simulink model "SPGF_FSK_0000_R2019b"  (R2019b)
settings: Solver=ode3  SolverName=ode4  StartTime=0.0  StopTime=1.4  FixedStep=50e-6/50  RelTol=1e-3  EnableMultiTasking=on
undefined symbols (not defined in the file): D11, Delta
libraries: powerlib x2544, powerlib_meascontrol x204, simulink x24
(part 3 of 33)

== system SPGF_FSK_0000_R2019b/TP21 ==
  Load : powerlib/Elements/Three-Phase Parallel RLC Load  Commented=on  LConnTagsString=A|B|C  Configuration=Y (grounded)  NominalVoltage=380  Vabc=[1e3 1e3 1e3]  Vabcp=[1e3 1e3 1e3]  NominalFrequency=50  UnbalancedPower=off  ActivePower=352800  InductivePower=158760  CapacitivePower=0  Pabc=[10e3 9e3 11e3]  QLabc=[100 90 110]  QCabc=[100 90 110]  Pabcp=[10e3 9e3 11e3]  QLabcp=[100 90 110]  QCabcp=[100 90 110]  Measurements=None  LoadType=constant PQ
  Nonlinear Load : Subsystem  Commented=on
  Nonlinear Load 3ph : Subsystem
  Q : Subsystem
  T : powerlib/Elements/Three-Phase Transformer (Two Windings)  Winding1Connection=Delta (D11)  Winding2Connection=Yg  CoreType=Three single-phase transformers  SetSaturation=on  Hysteresis=off  DataFile='hysteresis'  SetInitialFlux=off  Measurements=None  UNITS=pu  NominalPower=[630000, 50]  Winding1=[10250, 0.00603175, 0.02750000]  Winding2=[400.00, 0.00603175, 0.02750000]  Rm=504  Lm=58.8235  L0=2  Saturation=[0 0;0.01774 0.324129;0.0487637 0.61284;0.0980856 0.825118;0.2 1;0.309543 1.08024;0.652348 1.17344;2.0357 1.26115;6.0215 1.36094;12.4388 1.49469]  InitialFluxes=[-1.05034903009959 0.547738747303872 0.502610282795804]  BreakLoop=on  DiscreteSolver=Trapezoidal iterative  DataType=off  TransfoNumber=1
  Three-Phase Series RLC Load : powerlib/Elements/Three-Phase Series RLC Load  Commented=on  LConnTagsString=A|B|C  Configuration=Y (grounded)  NominalVoltage=380  Vabc=[1e3 1e3 1e3]  Vabcp=[1e3 1e3 1e3]  NominalFrequency=50  UnbalancedPower=off  ActivePower=352800  InductivePower=158760  CapacitivePower=0  Pabc=[10e3 9e3 11e3]  QLabc=[100 90 110]  QCabc=[100 90 110]  Pabcp=[10e3 9e3 11e3]  QLabcp=[100 90 110]  QCabcp=[100 90 110]  Measurements=None  LoadType=constant Z
  Three-Phase Series RLC Load1 : powerlib/Elements/Three-Phase Series RLC Load  LConnTagsString=A|B|C  Configuration=Y (grounded)  NominalVoltage=380  Vabc=[1e3 1e3 1e3]  Vabcp=[1e3 1e3 1e3]  NominalFrequency=50  UnbalancedPower=off  ActivePower=0.1*352800  InductivePower=0  CapacitivePower=0  Pabc=[10e3 9e3 11e3]  QLabc=[100 90 110]  QCabc=[100 90 110]  Pabcp=[10e3 9e3 11e3]  QLabcp=[100 90 110]  QCabcp=[100 90 110]  Measurements=None  LoadType=constant Z
  Three-Phase Series RLC Load2 : powerlib/Elements/Three-Phase Series RLC Load  LConnTagsString=A|B|C  Configuration=Y (grounded)  NominalVoltage=380  Vabc=[1e3 1e3 1e3]  Vabcp=[1e3 1e3 1e3]  NominalFrequency=50  UnbalancedPower=off  ActivePower=0.9*352800  InductivePower=158760  CapacitivePower=0  Pabc=[10e3 9e3 11e3]  QLabc=[100 90 110]  QCabc=[100 90 110]  Pabcp=[10e3 9e3 11e3]  QLabcp=[100 90 110]  QCabcp=[100 90 110]  Measurements=None  LoadType=constant Z
  A : PMIOPort  Side=Right
  B : PMIOPort  Port=2  Side=Right
  C : PMIOPort  Port=3  Side=Right
  connections:
  Three-Phase Series RLC Load/LConn1 -- Nonlinear Load/LConn1 -- Nonlinear Load 3ph/LConn1 -- T/RConn1 -- Load/LConn1 -- Three-Phase Series RLC Load2/LConn1 -- Three-Phase Series RLC Load1/LConn1
  Three-Phase Series RLC Load1/LConn2 -- Three-Phase Series RLC Load2/LConn2 -- Nonlinear Load/LConn2 -- Nonlinear Load 3ph/LConn2 -- Load/LConn2 -- T/RConn2 -- Three-Phase Series RLC Load/LConn2
  Three-Phase Series RLC Load1/LConn3 -- Three-Phase Series RLC Load2/LConn3 -- Nonlinear Load/LConn3 -- Nonlinear Load 3ph/LConn3 -- Load/LConn3 -- T/RConn3 -- Three-Phase Series RLC Load/LConn3
  Q/RConn3 -- C/RConn1
  Q/LConn2 -- T/LConn2
  Q/RConn1 -- A/RConn1
  Q/RConn2 -- B/RConn1
  Q/LConn1 -- T/LConn1
  Q/LConn3 -- T/LConn3

== system SPGF_FSK_0000_R2019b/TP22 ==
  Load : powerlib/Elements/Three-Phase Parallel RLC Load  Commented=on  LConnTagsString=A|B|C  Configuration=Y (grounded)  NominalVoltage=380  Vabc=[1e3 1e3 1e3]  Vabcp=[1e3 1e3 1e3]  NominalFrequency=50  UnbalancedPower=off  ActivePower=352800  InductivePower=158760  CapacitivePower=0  Pabc=[10e3 9e3 11e3]  QLabc=[100 90 110]  QCabc=[100 90 110]  Pabcp=[10e3 9e3 11e3]  QLabcp=[100 90 110]  QCabcp=[100 90 110]  Measurements=None  LoadType=constant PQ
  Nonlinear Load : Subsystem  Commented=on
  Nonlinear Load 3ph : Subsystem
  Q : Subsystem
  T : powerlib/Elements/Three-Phase Transformer (Two Windings)  Winding1Connection=Delta (D11)  Winding2Connection=Yg  CoreType=Three single-phase transformers  SetSaturation=on  Hysteresis=off  DataFile='hysteresis'  SetInitialFlux=off  Measurements=None  UNITS=pu  NominalPower=[630000, 50]  Winding1=[10250, 0.00603175, 0.02750000]  Winding2=[400.00, 0.00603175, 0.02750000]  Rm=504  Lm=58.8235  L0=2  Saturation=[0 0;0.01774 0.324129;0.0487637 0.61284;0.0980856 0.825118;0.2 1;0.309543 1.08024;0.652348 1.17344;2.0357 1.26115;6.0215 1.36094;12.4388 1.49469]  InitialFluxes=[-1.04995444167594 0.547468251609687 0.502486190066125]  BreakLoop=on  DiscreteSolver=Trapezoidal iterative  DataType=off  TransfoNumber=1
  Three-Phase Series RLC Load : powerlib/Elements/Three-Phase Series RLC Load  Commented=on  LConnTagsString=A|B|C  Configuration=Y (grounded)  NominalVoltage=380  Vabc=[1e3 1e3 1e3]  Vabcp=[1e3 1e3 1e3]  NominalFrequency=50  UnbalancedPower=off  ActivePower=352800  InductivePower=158760  CapacitivePower=0  Pabc=[10e3 9e3 11e3]  QLabc=[100 90 110]  QCabc=[100 90 110]  Pabcp=[10e3 9e3 11e3]  QLabcp=[100 90 110]  QCabcp=[100 90 110]  Measurements=None  LoadType=constant Z
  Three-Phase Series RLC Load1 : powerlib/Elements/Three-Phase Series RLC Load  LConnTagsString=A|B|C  Configuration=Y (grounded)  NominalVoltage=380  Vabc=[1e3 1e3 1e3]  Vabcp=[1e3 1e3 1e3]  NominalFrequency=50  UnbalancedPower=off  ActivePower=0.1*352800  InductivePower=0  CapacitivePower=0  Pabc=[10e3 9e3 11e3]  QLabc=[100 90 110]  QCabc=[100 90 110]  Pabcp=[10e3 9e3 11e3]  QLabcp=[100 90 110]  QCabcp=[100 90 110]  Measurements=None  LoadType=constant Z
  Three-Phase Series RLC Load2 : powerlib/Elements/Three-Phase Series RLC Load  LConnTagsString=A|B|C  Configuration=Y (grounded)  NominalVoltage=380  Vabc=[1e3 1e3 1e3]  Vabcp=[1e3 1e3 1e3]  NominalFrequency=50  UnbalancedPower=off  ActivePower=0.9*352800  InductivePower=158760  CapacitivePower=0  Pabc=[10e3 9e3 11e3]  QLabc=[100 90 110]  QCabc=[100 90 110]  Pabcp=[10e3 9e3 11e3]  QLabcp=[100 90 110]  QCabcp=[100 90 110]  Measurements=None  LoadType=constant Z
  A : PMIOPort  Side=Right
  B : PMIOPort  Port=2  Side=Right
  C : PMIOPort  Port=3  Side=Right
  connections:
  Q/LConn3 -- T/LConn3
  Q/LConn1 -- T/LConn1
  Q/RConn2 -- B/RConn1
  Q/RConn1 -- A/RConn1
  Q/LConn2 -- T/LConn2
  Q/RConn3 -- C/RConn1
  Three-Phase Series RLC Load1/LConn3 -- Three-Phase Series RLC Load2/LConn3 -- Nonlinear Load/LConn3 -- Nonlinear Load 3ph/LConn3 -- T/RConn3 -- Load/LConn3 -- Three-Phase Series RLC Load/LConn3
  Three-Phase Series RLC Load1/LConn2 -- Three-Phase Series RLC Load2/LConn2 -- Nonlinear Load/LConn2 -- Nonlinear Load 3ph/LConn2 -- Load/LConn2 -- T/RConn2 -- Three-Phase Series RLC Load/LConn2
  Three-Phase Series RLC Load/LConn1 -- Nonlinear Load/LConn1 -- Nonlinear Load 3ph/LConn1 -- Load/LConn1 -- T/RConn1 -- Three-Phase Series RLC Load2/LConn1 -- Three-Phase Series RLC Load1/LConn1

== system SPGF_FSK_0000_R2019b/TP31 ==
  Load : powerlib/Elements/Three-Phase Parallel RLC Load  Commented=on  LConnTagsString=A|B|C  Configuration=Y (grounded)  NominalVoltage=380  Vabc=[1e3 1e3 1e3]  Vabcp=[1e3 1e3 1e3]  NominalFrequency=50  UnbalancedPower=off  ActivePower=560000  InductivePower=252000  CapacitivePower=0  Pabc=[10e3 9e3 11e3]  QLabc=[100 90 110]  QCabc=[100 90 110]  Pabcp=[10e3 9e3 11e3]  QLabcp=[100 90 110]  QCabcp=[100 90 110]  Measurements=None  LoadType=constant PQ
  Nonlinear Load : Subsystem  Commented=on
  Nonlinear Load 3ph : Subsystem
  Q : Subsystem
  T : powerlib/Elements/Three-Phase Transformer (Two Windings)  Winding1Connection=Y  Winding2Connection=Yg  CoreType=Three single-phase transformers  SetSaturation=on  Hysteresis=off  DataFile='hysteresis'  SetInitialFlux=off  Measurements=None  UNITS=pu  NominalPower=[1000000, 50]  Winding1=[10250, 0.00610000, 0.02750000]  Winding2=[400.00, 0.00610000, 0.02750000]  Rm=526.316  Lm=58.8235  L0=2  Saturation=[0 0;0.01774 0.324129;0.0487637 0.61284;0.0980856 0.825118;0.2 1;0.309543 1.08024;0.652348 1.17344;2.0357 1.26115;6.0215 1.36094;12.4388 1.49469]  InitialFluxes=[-0.919016130821894 0.0257026532083102 0.893313477613749]  BreakLoop=on  DiscreteSolver=Trapezoidal iterative  DataType=off  TransfoNumber=1
  Three-Phase Series RLC Load : powerlib/Elements/Three-Phase Series RLC Load  Commented=on  LConnTagsString=A|B|C  Configuration=Y (grounded)  NominalVoltage=380  Vabc=[1e3 1e3 1e3]  Vabcp=[1e3 1e3 1e3]  NominalFrequency=50  UnbalancedPower=off  ActivePower=560000  InductivePower=252000  CapacitivePower=0  Pabc=[10e3 9e3 11e3]  QLabc=[100 90 110]  QCabc=[100 90 110]  Pabcp=[10e3 9e3 11e3]  QLabcp=[100 90 110]  QCabcp=[100 90 110]  Measurements=None  LoadType=constant Z
  Three-Phase Series RLC Load1 : powerlib/Elements/Three-Phase Series RLC Load  LConnTagsString=A|B|C  Configuration=Y (grounded)  NominalVoltage=380  Vabc=[1e3 1e3 1e3]  Vabcp=[1e3 1e3 1e3]  NominalFrequency=50  UnbalancedPower=off  ActivePower=0.1*560000  InductivePower=0  CapacitivePower=0  Pabc=[10e3 9e3 11e3]  QLabc=[100 90 110]  QCabc=[100 90 110]  Pabcp=[10e3 9e3 11e3]  QLabcp=[100 90 110]  QCabcp=[100 90 110]  Measurements=None  LoadType=constant Z
  Three-Phase Series RLC Load2 : powerlib/Elements/Three-Phase Series RLC Load  LConnTagsString=A|B|C  Configuration=Y (grounded)  NominalVoltage=380  Vabc=[1e3 1e3 1e3]  Vabcp=[1e3 1e3 1e3]  NominalFrequency=50  UnbalancedPower=off  ActivePower=0.9*560000  InductivePower=252000  CapacitivePower=0  Pabc=[10e3 9e3 11e3]  QLabc=[100 90 110]  QCabc=[100 90 110]  Pabcp=[10e3 9e3 11e3]  QLabcp=[100 90 110]  QCabcp=[100 90 110]  Measurements=None  LoadType=constant Z
  A : PMIOPort  Side=Right
  B : PMIOPort  Port=2  Side=Right
  C : PMIOPort  Port=3  Side=Right
  connections:
  Three-Phase Series RLC Load/LConn1 -- Nonlinear Load/LConn1 -- Nonlinear Load 3ph/LConn1 -- T/RConn1 -- Load/LConn1 -- Three-Phase Series RLC Load2/LConn1 -- Three-Phase Series RLC Load1/LConn1
  Three-Phase Series RLC Load1/LConn2 -- Three-Phase Series RLC Load2/LConn2 -- Nonlinear Load/LConn2 -- Nonlinear Load 3ph/LConn2 -- T/RConn2 -- Load/LConn2 -- Three-Phase Series RLC Load/LConn2
  Three-Phase Series RLC Load1/LConn3 -- Three-Phase Series RLC Load2/LConn3 -- Nonlinear Load/LConn3 -- Nonlinear Load 3ph/LConn3 -- T/RConn3 -- Load/LConn3 -- Three-Phase Series RLC Load/LConn3
  Q/RConn3 -- C/RConn1
  Q/LConn2 -- T/LConn2
  Q/RConn1 -- A/RConn1
  Q/RConn2 -- B/RConn1
  Q/LConn1 -- T/LConn1
  Q/LConn3 -- T/LConn3

== system SPGF_FSK_0000_R2019b/TP321 ==
  Load : powerlib/Elements/Three-Phase Parallel RLC Load  Commented=on  LConnTagsString=A|B|C  Configuration=Y (grounded)  NominalVoltage=380  Vabc=[1e3 1e3 1e3]  Vabcp=[1e3 1e3 1e3]  NominalFrequency=50  UnbalancedPower=off  ActivePower=352800  InductivePower=158760  CapacitivePower=0  Pabc=[10e3 9e3 11e3]  QLabc=[100 90 110]  QCabc=[100 90 110]  Pabcp=[10e3 9e3 11e3]  QLabcp=[100 90 110]  QCabcp=[100 90 110]  Measurements=None  LoadType=constant PQ
  Nonlinear Load : Subsystem  Commented=on
  Nonlinear Load 3ph : Subsystem
  Q : Subsystem
  T : powerlib/Elements/Three-Phase Transformer (Two Windings)  Winding1Connection=Delta (D11)  Winding2Connection=Yg  CoreType=Three single-phase transformers  SetSaturation=on  Hysteresis=off  DataFile='hysteresis'  SetInitialFlux=off  Measurements=None  UNITS=pu  NominalPower=[630000, 50]  Winding1=[10250, 0.00603175, 0.02750000]  Winding2=[400.00, 0.00603175, 0.02750000]  Rm=504  Lm=58.8235  L0=2  Saturation=[0 0;0.01774 0.324129;0.0487637 0.61284;0.0980856 0.825118;0.2 1;0.309543 1.08024;0.652348 1.17344;2.0357 1.26115;6.0215 1.36094;12.4388 1.49469]  InitialFluxes=[-1.04481909477767 0.544399254332123 0.500419840445666]  BreakLoop=on  DiscreteSolver=Trapezoidal iterative  DataType=off  TransfoNumber=1
  Three-Phase Series RLC Load : powerlib/Elements/Three-Phase Series RLC Load  Commented=on  LConnTagsString=A|B|C  Configuration=Y (grounded)  NominalVoltage=380  Vabc=[1e3 1e3 1e3]  Vabcp=[1e3 1e3 1e3]  NominalFrequency=50  UnbalancedPower=off  ActivePower=352800  InductivePower=158760  CapacitivePower=0  Pabc=[10e3 9e3 11e3]  QLabc=[100 90 110]  QCabc=[100 90 110]  Pabcp=[10e3 9e3 11e3]  QLabcp=[100 90 110]  QCabcp=[100 90 110]  Measurements=None  LoadType=constant Z
  Three-Phase Series RLC Load1 : powerlib/Elements/Three-Phase Series RLC Load  LConnTagsString=A|B|C  Configuration=Y (grounded)  NominalVoltage=380  Vabc=[1e3 1e3 1e3]  Vabcp=[1e3 1e3 1e3]  NominalFrequency=50  UnbalancedPower=off  ActivePower=0.1*352800  InductivePower=0  CapacitivePower=0  Pabc=[10e3 9e3 11e3]  QLabc=[100 90 110]  QCabc=[100 90 110]  Pabcp=[10e3 9e3 11e3]  QLabcp=[100 90 110]  QCabcp=[100 90 110]  Measurements=None  LoadType=constant Z
  Three-Phase Series RLC Load2 : powerlib/Elements/Three-Phase Series RLC Load  LConnTagsString=A|B|C  Configuration=Y (grounded)  NominalVoltage=380  Vabc=[1e3 1e3 1e3]  Vabcp=[1e3 1e3 1e3]  NominalFrequency=50  UnbalancedPower=off  ActivePower=0.9*352800  InductivePower=158760  CapacitivePower=0  Pabc=[10e3 9e3 11e3]  QLabc=[100 90 110]  QCabc=[100 90 110]  Pabcp=[10e3 9e3 11e3]  QLabcp=[100 90 110]  QCabcp=[100 90 110]  Measurements=None  LoadType=constant Z
  A : PMIOPort  Side=Right
  B : PMIOPort  Port=2  Side=Right
  C : PMIOPort  Port=3  Side=Right
  connections:
  Q/LConn3 -- T/LConn3
  Q/LConn1 -- T/LConn1
  Q/RConn2 -- B/RConn1
  Q/RConn1 -- A/RConn1
  Q/LConn2 -- T/LConn2
  Q/RConn3 -- C/RConn1
  Three-Phase Series RLC Load1/LConn3 -- Three-Phase Series RLC Load2/LConn3 -- Nonlinear Load/LConn3 -- Nonlinear Load 3ph/LConn3 -- T/RConn3 -- Load/LConn3 -- Three-Phase Series RLC Load/LConn3
  Three-Phase Series RLC Load1/LConn2 -- Three-Phase Series RLC Load2/LConn2 -- Nonlinear Load/LConn2 -- Nonlinear Load 3ph/LConn2 -- Load/LConn2 -- T/RConn2 -- Three-Phase Series RLC Load/LConn2
  Three-Phase Series RLC Load/LConn1 -- Nonlinear Load/LConn1 -- Nonlinear Load 3ph/LConn1 -- Load/LConn1 -- T/RConn1 -- Three-Phase Series RLC Load2/LConn1 -- Three-Phase Series RLC Load1/LConn1

== system SPGF_FSK_0000_R2019b/TP322 ==
  Load : powerlib/Elements/Three-Phase Parallel RLC Load  Commented=on  LConnTagsString=A|B|C  Configuration=Y (grounded)  NominalVoltage=380  Vabc=[1e3 1e3 1e3]  Vabcp=[1e3 1e3 1e3]  NominalFrequency=50  UnbalancedPower=off  ActivePower=352800  InductivePower=158760  CapacitivePower=0  Pabc=[10e3 9e3 11e3]  QLabc=[100 90 110]  QCabc=[100 90 110]  Pabcp=[10e3 9e3 11e3]  QLabcp=[100 90 110]  QCabcp=[100 90 110]  Measurements=None  LoadType=constant PQ
  Nonlinear Load : Subsystem  Commented=on
  Nonlinear Load 3ph : Subsystem
  Q : Subsystem
  T : powerlib/Elements/Three-Phase Transformer (Two Windings)  Winding1Connection=Delta (D11)  Winding2Connection=Yg  CoreType=Three single-phase transformers  SetSaturation=on  Hysteresis=off  DataFile='hysteresis'  SetInitialFlux=off  Measurements=None  UNITS=pu  NominalPower=[630000, 50]  Winding1=[10250, 0.00603175, 0.02750000]  Winding2=[400.00, 0.00603175, 0.02750000]  Rm=504  Lm=58.8235  L0=2  Saturation=[0 0;0.01774 0.324129;0.0487637 0.61284;0.0980856 0.825118;0.2 1;0.309543 1.08024;0.652348 1.17344;2.0357 1.26115;6.0215 1.36094;12.4388 1.49469]  InitialFluxes=[-1.0448190947778 0.544399254332092 0.500419840445633]  BreakLoop=on  DiscreteSolver=Trapezoidal iterative  DataType=off  TransfoNumber=1
  Three-Phase Series RLC Load : powerlib/Elements/Three-Phase Series RLC Load  Commented=on  LConnTagsString=A|B|C  Configuration=Y (grounded)  NominalVoltage=380  Vabc=[1e3 1e3 1e3]  Vabcp=[1e3 1e3 1e3]  NominalFrequency=50  UnbalancedPower=off  ActivePower=352800  InductivePower=158760  CapacitivePower=0  Pabc=[10e3 9e3 11e3]  QLabc=[100 90 110]  QCabc=[100 90 110]  Pabcp=[10e3 9e3 11e3]  QLabcp=[100 90 110]  QCabcp=[100 90 110]  Measurements=None  LoadType=constant Z
  Three-Phase Series RLC Load1 : powerlib/Elements/Three-Phase Series RLC Load  LConnTagsString=A|B|C  Configuration=Y (grounded)  NominalVoltage=380  Vabc=[1e3 1e3 1e3]  Vabcp=[1e3 1e3 1e3]  NominalFrequency=50  UnbalancedPower=off  ActivePower=0.1*352800  InductivePower=0  CapacitivePower=0  Pabc=[10e3 9e3 11e3]  QLabc=[100 90 110]  QCabc=[100 90 110]  Pabcp=[10e3 9e3 11e3]  QLabcp=[100 90 110]  QCabcp=[100 90 110]  Measurements=None  LoadType=constant Z
  Three-Phase Series RLC Load2 : powerlib/Elements/Three-Phase Series RLC Load  LConnTagsString=A|B|C  Configuration=Y (grounded)  NominalVoltage=380  Vabc=[1e3 1e3 1e3]  Vabcp=[1e3 1e3 1e3]  NominalFrequency=50  UnbalancedPower=off  ActivePower=0.9*352800  InductivePower=158760  CapacitivePower=0  Pabc=[10e3 9e3 11e3]  QLabc=[100 90 110]  QCabc=[100 90 110]  Pabcp=[10e3 9e3 11e3]  QLabcp=[100 90 110]  QCabcp=[100 90 110]  Measurements=None  LoadType=constant Z
  A : PMIOPort  Side=Right
  B : PMIOPort  Port=2  Side=Right
  C : PMIOPort  Port=3  Side=Right
  connections:
  Three-Phase Series RLC Load/LConn1 -- Nonlinear Load/LConn1 -- Nonlinear Load 3ph/LConn1 -- Load/LConn1 -- T/RConn1 -- Three-Phase Series RLC Load2/LConn1 -- Three-Phase Series RLC Load1/LConn1
  Three-Phase Series RLC Load1/LConn2 -- Three-Phase Series RLC Load2/LConn2 -- Nonlinear Load/LConn2 -- Nonlinear Load 3ph/LConn2 -- T/RConn2 -- Load/LConn2 -- Three-Phase Series RLC Load/LConn2
  Three-Phase Series RLC Load1/LConn3 -- Three-Phase Series RLC Load2/LConn3 -- Nonlinear Load/LConn3 -- Nonlinear Load 3ph/LConn3 -- T/RConn3 -- Load/LConn3 -- Three-Phase Series RLC Load/LConn3
  Q/RConn3 -- C/RConn1
  Q/LConn2 -- T/LConn2
  Q/RConn1 -- A/RConn1
  Q/RConn2 -- B/RConn1
  Q/LConn1 -- T/LConn1
  Q/LConn3 -- T/LConn3

== system SPGF_FSK_0000_R2019b/TP33 ==
  Load : powerlib/Elements/Three-Phase Parallel RLC Load  Commented=on  LConnTagsString=A|B|C  Configuration=Y (grounded)  NominalVoltage=380  Vabc=[1e3 1e3 1e3]  Vabcp=[1e3 1e3 1e3]  NominalFrequency=50  UnbalancedPower=off  ActivePower=560000  InductivePower=252000  CapacitivePower=0  Pabc=[10e3 9e3 11e3]  QLabc=[100 90 110]  QCabc=[100 90 110]  Pabcp=[10e3 9e3 11e3]  QLabcp=[100 90 110]  QCabcp=[100 90 110]  Measurements=None  LoadType=constant PQ
  Nonlinear Load : Subsystem  Commented=on
  Nonlinear Load 3ph : Subsystem
  Q : Subsystem
  T : powerlib/Elements/Three-Phase Transformer (Two Windings)  Winding1Connection=Y  Winding2Connection=Yg  CoreType=Three single-phase transformers  SetSaturation=on  Hysteresis=off  DataFile='hysteresis'  SetInitialFlux=off  Measurements=None  UNITS=pu  NominalPower=[1000000, 50]  Winding1=[10250, 0.00610000, 0.02750000]  Winding2=[400.00, 0.00610000, 0.02750000]  Rm=526.316  Lm=58.8235  L0=2  Saturation=[0 0;0.01774 0.324129;0.0487637 0.61284;0.0980856 0.825118;0.2 1;0.309543 1.08024;0.652348 1.17344;2.0357 1.26115;6.0215 1.36094;12.4388 1.49469]  InitialFluxes=[-0.916567668392243 0.025179277852983 0.891388390539228]  BreakLoop=on  DiscreteSolver=Trapezoidal iterative  DataType=off  TransfoNumber=1
  Three-Phase Series RLC Load : powerlib/Elements/Three-Phase Series RLC Load  Commented=on  LConnTagsString=A|B|C  Configuration=Y (grounded)  NominalVoltage=380  Vabc=[1e3 1e3 1e3]  Vabcp=[1e3 1e3 1e3]  NominalFrequency=50  UnbalancedPower=off  ActivePower=560000  InductivePower=252000  CapacitivePower=0  Pabc=[10e3 9e3 11e3]  QLabc=[100 90 110]  QCabc=[100 90 110]  Pabcp=[10e3 9e3 11e3]  QLabcp=[100 90 110]  QCabcp=[100 90 110]  Measurements=None  LoadType=constant Z
  Three-Phase Series RLC Load1 : powerlib/Elements/Three-Phase Series RLC Load  LConnTagsString=A|B|C  Configuration=Y (grounded)  NominalVoltage=380  Vabc=[1e3 1e3 1e3]  Vabcp=[1e3 1e3 1e3]  NominalFrequency=50  UnbalancedPower=off  ActivePower=0.1*560000  InductivePower=0  CapacitivePower=0  Pabc=[10e3 9e3 11e3]  QLabc=[100 90 110]  QCabc=[100 90 110]  Pabcp=[10e3 9e3 11e3]  QLabcp=[100 90 110]  QCabcp=[100 90 110]  Measurements=None  LoadType=constant Z
  Three-Phase Series RLC Load2 : powerlib/Elements/Three-Phase Series RLC Load  LConnTagsString=A|B|C  Configuration=Y (grounded)  NominalVoltage=380  Vabc=[1e3 1e3 1e3]  Vabcp=[1e3 1e3 1e3]  NominalFrequency=50  UnbalancedPower=off  ActivePower=0.9*560000  InductivePower=252000  CapacitivePower=0  Pabc=[10e3 9e3 11e3]  QLabc=[100 90 110]  QCabc=[100 90 110]  Pabcp=[10e3 9e3 11e3]  QLabcp=[100 90 110]  QCabcp=[100 90 110]  Measurements=None  LoadType=constant Z
  A : PMIOPort  Side=Right
  B : PMIOPort  Port=2  Side=Right
  C : PMIOPort  Port=3  Side=Right
  connections:
  Q/LConn3 -- T/LConn3
  Q/LConn1 -- T/LConn1
  Q/RConn2 -- B/RConn1
  Q/RConn1 -- A/RConn1
  Q/LConn2 -- T/LConn2
  Q/RConn3 -- C/RConn1
  Three-Phase Series RLC Load1/LConn3 -- Three-Phase Series RLC Load2/LConn3 -- Nonlinear Load/LConn3 -- Nonlinear Load 3ph/LConn3 -- T/RConn3 -- Load/LConn3 -- Three-Phase Series RLC Load/LConn3
  Three-Phase Series RLC Load1/LConn2 -- Three-Phase Series RLC Load2/LConn2 -- Nonlinear Load/LConn2 -- Nonlinear Load 3ph/LConn2 -- Load/LConn2 -- T/RConn2 -- Three-Phase Series RLC Load/LConn2
  Three-Phase Series RLC Load/LConn1 -- Nonlinear Load/LConn1 -- Nonlinear Load 3ph/LConn1 -- Load/LConn1 -- T/RConn1 -- Three-Phase Series RLC Load2/LConn1 -- Three-Phase Series RLC Load1/LConn1

== system SPGF_FSK_0000_R2019b/TP34 ==
  Load : powerlib/Elements/Three-Phase Parallel RLC Load  Commented=on  LConnTagsString=A|B|C  Configuration=Y (grounded)  NominalVoltage=380  Vabc=[1e3 1e3 1e3]  Vabcp=[1e3 1e3 1e3]  NominalFrequency=50  UnbalancedPower=off  ActivePower=352800  InductivePower=158760  CapacitivePower=0  Pabc=[10e3 9e3 11e3]  QLabc=[100 90 110]  QCabc=[100 90 110]  Pabcp=[10e3 9e3 11e3]  QLabcp=[100 90 110]  QCabcp=[100 90 110]  Measurements=None  LoadType=constant PQ
  Nonlinear Load : Subsystem  Commented=on
  Nonlinear Load 3ph : Subsystem
  Q : Subsystem
  T : powerlib/Elements/Three-Phase Transformer (Two Windings)  Winding1Connection=Delta (D11)  Winding2Connection=Yg  CoreType=Three single-phase transformers  SetSaturation=on  Hysteresis=off  DataFile='hysteresis'  SetInitialFlux=off  Measurements=None  UNITS=pu  NominalPower=[630000, 50]  Winding1=[10250, 0.00603175, 0.02750000]  Winding2=[400.00, 0.00603175, 0.02750000]  Rm=504  Lm=58.8235  L0=2  Saturation=[0 0;0.01774 0.324129;0.0487637 0.61284;0.0980856 0.825118;0.2 1;0.309543 1.08024;0.652348 1.17344;2.0357 1.26115;6.0215 1.36094;12.4388 1.49469]  InitialFluxes=[-1.04232437769437 0.542559009201154 0.499765368493118]  BreakLoop=on  DiscreteSolver=Trapezoidal iterative  DataType=off  TransfoNumber=1
  Three-Phase Series RLC Load : powerlib/Elements/Three-Phase Series RLC Load  Commented=on  LConnTagsString=A|B|C  Configuration=Y (grounded)  NominalVoltage=380  Vabc=[1e3 1e3 1e3]  Vabcp=[1e3 1e3 1e3]  NominalFrequency=50  UnbalancedPower=off  ActivePower=352800  InductivePower=158760  CapacitivePower=0  Pabc=[10e3 9e3 11e3]  QLabc=[100 90 110]  QCabc=[100 90 110]  Pabcp=[10e3 9e3 11e3]  QLabcp=[100 90 110]  QCabcp=[100 90 110]  Measurements=None  LoadType=constant Z
  Three-Phase Series RLC Load1 : powerlib/Elements/Three-Phase Series RLC Load  LConnTagsString=A|B|C  Configuration=Y (grounded)  NominalVoltage=380  Vabc=[1e3 1e3 1e3]  Vabcp=[1e3 1e3 1e3]  NominalFrequency=50  UnbalancedPower=off  ActivePower=0.1*352800  InductivePower=0  CapacitivePower=0  Pabc=[10e3 9e3 11e3]  QLabc=[100 90 110]  QCabc=[100 90 110]  Pabcp=[10e3 9e3 11e3]  QLabcp=[100 90 110]  QCabcp=[100 90 110]  Measurements=None  LoadType=constant Z
  Three-Phase Series RLC Load2 : powerlib/Elements/Three-Phase Series RLC Load  LConnTagsString=A|B|C  Configuration=Y (grounded)  NominalVoltage=380  Vabc=[1e3 1e3 1e3]  Vabcp=[1e3 1e3 1e3]  NominalFrequency=50  UnbalancedPower=off  ActivePower=0.9*352800  InductivePower=158760  CapacitivePower=0  Pabc=[10e3 9e3 11e3]  QLabc=[100 90 110]  QCabc=[100 90 110]  Pabcp=[10e3 9e3 11e3]  QLabcp=[100 90 110]  QCabcp=[100 90 110]  Measurements=None  LoadType=constant Z
  A : PMIOPort  Side=Right
  B : PMIOPort  Port=2  Side=Right
  C : PMIOPort  Port=3  Side=Right
  connections:
  Three-Phase Series RLC Load2/LConn1 -- Three-Phase Series RLC Load1/LConn1 -- Three-Phase Series RLC Load/LConn1 -- Nonlinear Load/LConn1 -- Nonlinear Load 3ph/LConn1 -- Load/LConn1 -- T/RConn1
  Three-Phase Series RLC Load2/LConn2 -- Three-Phase Series RLC Load1/LConn2 -- Three-Phase Series RLC Load/LConn2 -- Nonlinear Load/LConn2 -- Nonlinear Load 3ph/LConn2 -- Load/LConn2 -- T/RConn2
  Three-Phase Series RLC Load1/LConn3 -- Three-Phase Series RLC Load2/LConn3 -- Three-Phase Series RLC Load/LConn3 -- Load/LConn3 -- T/RConn3 -- Nonlinear Load/LConn3 -- Nonlinear Load 3ph/LConn3
  Q/RConn3 -- C/RConn1
  Q/LConn2 -- T/LConn2
  Q/RConn1 -- A/RConn1
  Q/RConn2 -- B/RConn1
  Q/LConn1 -- T/LConn1
  Q/LConn3 -- T/LConn3

== system SPGF_FSK_0000_R2019b/TP35 ==
  Load : powerlib/Elements/Three-Phase Parallel RLC Load  Commented=on  LConnTagsString=A|B|C  Configuration=Y (grounded)  NominalVoltage=380  Vabc=[1e3 1e3 1e3]  Vabcp=[1e3 1e3 1e3]  NominalFrequency=50  UnbalancedPower=off  ActivePower=224000  InductivePower=100800  CapacitivePower=0  Pabc=[10e3 9e3 11e3]  QLabc=[100 90 110]  QCabc=[100 90 110]  Pabcp=[10e3 9e3 11e3]  QLabcp=[100 90 110]  QCabcp=[100 90 110]  Measurements=None  LoadType=constant PQ
  Nonlinear Load : Subsystem  Commented=on
  Nonlinear Load 3ph : Subsystem
  Q : Subsystem
  T : powerlib/Elements/Three-Phase Transformer (Two Windings)  Winding1Connection=Y  Winding2Connection=Yg  CoreType=Three single-phase transformers  SetSaturation=on  Hysteresis=off  DataFile='hysteresis'  SetInitialFlux=off  Measurements=None  UNITS=pu  NominalPower=[400000, 50]  Winding1=[10250, 0.00687500, 0.02250000]  Winding2=[400.00, 0.00687500, 0.02250000]  Rm=444.444  Lm=55.5556  L0=2  Saturation=[0 0;0.01774 0.324129;0.0487637 0.61284;0.0980856 0.825118;0.2 1;0.309543 1.08024;0.652348 1.17344;2.0357 1.26115;6.0215 1.36094;12.4388 1.49469]  InitialFluxes=[-0.913549221158618 0.0211591996653002 0.892390021493428]  BreakLoop=on  DiscreteSolver=Trapezoidal iterative  DataType=off  TransfoNumber=1
  Three-Phase Series RLC Load : powerlib/Elements/Three-Phase Series RLC Load  Commented=on  LConnTagsString=A|B|C  Configuration=Y (grounded)  NominalVoltage=380  Vabc=[1e3 1e3 1e3]  Vabcp=[1e3 1e3 1e3]  NominalFrequency=50  UnbalancedPower=off  ActivePower=224000  InductivePower=100800  CapacitivePower=0  Pabc=[10e3 9e3 11e3]  QLabc=[100 90 110]  QCabc=[100 90 110]  Pabcp=[10e3 9e3 11e3]  QLabcp=[100 90 110]  QCabcp=[100 90 110]  Measurements=None  LoadType=constant Z
  Three-Phase Series RLC Load1 : powerlib/Elements/Three-Phase Series RLC Load  LConnTagsString=A|B|C  Configuration=Y (grounded)  NominalVoltage=380  Vabc=[1e3 1e3 1e3]  Vabcp=[1e3 1e3 1e3]  NominalFrequency=50  UnbalancedPower=off  ActivePower=0.1*224000  InductivePower=0  CapacitivePower=0  Pabc=[10e3 9e3 11e3]  QLabc=[100 90 110]  QCabc=[100 90 110]  Pabcp=[10e3 9e3 11e3]  QLabcp=[100 90 110]  QCabcp=[100 90 110]  Measurements=None  LoadType=constant Z
  Three-Phase Series RLC Load2 : powerlib/Elements/Three-Phase Series RLC Load  LConnTagsString=A|B|C  Configuration=Y (grounded)  NominalVoltage=380  Vabc=[1e3 1e3 1e3]  Vabcp=[1e3 1e3 1e3]  NominalFrequency=50  UnbalancedPower=off  ActivePower=0.9*224000  InductivePower=100800  CapacitivePower=0  Pabc=[10e3 9e3 11e3]  QLabc=[100 90 110]  QCabc=[100 90 110]  Pabcp=[10e3 9e3 11e3]  QLabcp=[100 90 110]  QCabcp=[100 90 110]  Measurements=None  LoadType=constant Z
  A : PMIOPort  Side=Right
  B : PMIOPort  Port=2  Side=Right
  C : PMIOPort  Port=3  Side=Right
  connections:
  Q/LConn3 -- T/LConn3
  Q/LConn1 -- T/LConn1
  Q/RConn2 -- B/RConn1
  Q/RConn1 -- A/RConn1
  Q/LConn2 -- T/LConn2
  Q/RConn3 -- C/RConn1
  Three-Phase Series RLC Load1/LConn3 -- Three-Phase Series RLC Load2/LConn3 -- Nonlinear Load/LConn3 -- Nonlinear Load 3ph/LConn3 -- T/RConn3 -- Load/LConn3 -- Three-Phase Series RLC Load/LConn3
  Three-Phase Series RLC Load1/LConn2 -- Three-Phase Series RLC Load2/LConn2 -- Nonlinear Load/LConn2 -- Nonlinear Load 3ph/LConn2 -- T/RConn2 -- Load/LConn2 -- Three-Phase Series RLC Load/LConn2
  Three-Phase Series RLC Load/LConn1 -- Nonlinear Load/LConn1 -- Nonlinear Load 3ph/LConn1 -- Load/LConn1 -- T/RConn1 -- Three-Phase Series RLC Load2/LConn1 -- Three-Phase Series RLC Load1/LConn1

== system SPGF_FSK_0000_R2019b/TP41 ==
  Load : powerlib/Elements/Three-Phase Parallel RLC Load  Commented=on  LConnTagsString=A|B|C  Configuration=Y (grounded)  NominalVoltage=380  Vabc=[1e3 1e3 1e3]  Vabcp=[1e3 1e3 1e3]  NominalFrequency=50  UnbalancedPower=off  ActivePower=352800  InductivePower=158760  CapacitivePower=0  Pabc=[10e3 9e3 11e3]  QLabc=[100 90 110]  QCabc=[100 90 110]  Pabcp=[10e3 9e3 11e3]  QLabcp=[100 90 110]  QCabcp=[100 90 110]  Measurements=None  LoadType=constant PQ
  Nonlinear Load : Subsystem  Commented=on
  Nonlinear Load 3ph : Subsystem
  Q : Subsystem
  T : powerlib/Elements/Three-Phase Transformer (Two Windings)  Winding1Connection=Delta (D11)  Winding2Connection=Yg  CoreType=Three single-phase transformers  SetSaturation=on  Hysteresis=off  DataFile='hysteresis'  SetInitialFlux=off  Measurements=None  UNITS=pu  NominalPower=[630000, 50]  Winding1=[10250, 0.00603175, 0.02750000]  Winding2=[400.00, 0.00603175, 0.02750000]  Rm=504  Lm=58.8235  L0=2  Saturation=[0 0;0.01774 0.324129;0.0487637 0.61284;0.0980856 0.825118;0.2 1;0.309543 1.08024;0.652348 1.17344;2.0357 1.26115;6.0215 1.36094;12.4388 1.49469]  InitialFluxes=[-1.0503661048076 0.547751977522492 0.502614127285616]  BreakLoop=on  DiscreteSolver=Trapezoidal iterative  DataType=off  TransfoNumber=1
  Three-Phase Series RLC Load : powerlib/Elements/Three-Phase Series RLC Load  Commented=on  LConnTagsString=A|B|C  Configuration=Y (grounded)  NominalVoltage=380  Vabc=[1e3 1e3 1e3]  Vabcp=[1e3 1e3 1e3]  NominalFrequency=50  UnbalancedPower=off  ActivePower=352800  InductivePower=158760  CapacitivePower=0  Pabc=[10e3 9e3 11e3]  QLabc=[100 90 110]  QCabc=[100 90 110]  Pabcp=[10e3 9e3 11e3]  QLabcp=[100 90 110]  QCabcp=[100 90 110]  Measurements=None  LoadType=constant Z
  Three-Phase Series RLC Load1 : powerlib/Elements/Three-Phase Series RLC Load  LConnTagsString=A|B|C  Configuration=Y (grounded)  NominalVoltage=380  Vabc=[1e3 1e3 1e3]  Vabcp=[1e3 1e3 1e3]  NominalFrequency=50  UnbalancedPower=off  ActivePower=0.1*352800  InductivePower=0  CapacitivePower=0  Pabc=[10e3 9e3 11e3]  QLabc=[100 90 110]  QCabc=[100 90 110]  Pabcp=[10e3 9e3 11e3]  QLabcp=[100 90 110]  QCabcp=[100 90 110]  Measurements=None  LoadType=constant Z
  Three-Phase Series RLC Load2 : powerlib/Elements/Three-Phase Series RLC Load  LConnTagsString=A|B|C  Configuration=Y (grounded)  NominalVoltage=380  Vabc=[1e3 1e3 1e3]  Vabcp=[1e3 1e3 1e3]  NominalFrequency=50  UnbalancedPower=off  ActivePower=0.9*352800  InductivePower=158760  CapacitivePower=0  Pabc=[10e3 9e3 11e3]  QLabc=[100 90 110]  QCabc=[100 90 110]  Pabcp=[10e3 9e3 11e3]  QLabcp=[100 90 110]  QCabcp=[100 90 110]  Measurements=None  LoadType=constant Z
  A : PMIOPort  Side=Right
  B : PMIOPort  Port=2  Side=Right
  C : PMIOPort  Port=3  Side=Right
  connections:
  Three-Phase Series RLC Load2/LConn1 -- Three-Phase Series RLC Load1/LConn1 -- Nonlinear Load/LConn1 -- Nonlinear Load 3ph/LConn1 -- Load/LConn1 -- T/RConn1 -- Three-Phase Series RLC Load/LConn1
  Three-Phase Series RLC Load2/LConn2 -- Three-Phase Series RLC Load1/LConn2 -- Nonlinear Load/LConn2 -- Nonlinear Load 3ph/LConn2 -- T/RConn2 -- Load/LConn2 -- Three-Phase Series RLC Load/LConn2
  Three-Phase Series RLC Load2/LConn3 -- Three-Phase Series RLC Load1/LConn3 -- Nonlinear Load/LConn3 -- Nonlinear Load 3ph/LConn3 -- T/RConn3 -- Load/LConn3 -- Three-Phase Series RLC Load/LConn3
  Q/RConn3 -- C/RConn1
  Q/LConn2 -- T/LConn2
  Q/RConn1 -- A/RConn1
  Q/RConn2 -- B/RConn1
  Q/LConn1 -- T/LConn1
  Q/LConn3 -- T/LConn3

== system SPGF_FSK_0000_R2019b/TP42 ==
  Load : powerlib/Elements/Three-Phase Parallel RLC Load  Commented=on  LConnTagsString=A|B|C  Configuration=Y (grounded)  NominalVoltage=380  Vabc=[1e3 1e3 1e3]  Vabcp=[1e3 1e3 1e3]  NominalFrequency=50  UnbalancedPower=off  ActivePower=352800  InductivePower=158760  CapacitivePower=0  Pabc=[10e3 9e3 11e3]  QLabc=[100 90 110]  QCabc=[100 90 110]  Pabcp=[10e3 9e3 11e3]  QLabcp=[100 90 110]  QCabcp=[100 90 110]  Measurements=None  LoadType=constant PQ
  Nonlinear Load : Subsystem  Commented=on
  Nonlinear Load 3ph : Subsystem
  Q : Subsystem
  T : powerlib/Elements/Three-Phase Transformer (Two Windings)  Winding1Connection=Delta (D11)  Winding2Connection=Yg  CoreType=Three single-phase transformers  SetSaturation=on  Hysteresis=off  DataFile='hysteresis'  SetInitialFlux=off  Measurements=None  UNITS=pu  NominalPower=[630000, 50]  Winding1=[10250, 0.00603175, 0.02750000]  Winding2=[400.00, 0.00603175, 0.02750000]  Rm=504  Lm=58.8235  L0=2  Saturation=[0 0;0.01774 0.324129;0.0487637 0.61284;0.0980856 0.825118;0.2 1;0.309543 1.08024;0.652348 1.17344;2.0357 1.26115;6.0215 1.36094;12.4388 1.49469]  InitialFluxes=[-1.04929135905229 0.547022493837419 0.502268865215033]  BreakLoop=on  DiscreteSolver=Trapezoidal iterative  DataType=off  TransfoNumber=1
  Three-Phase Series RLC Load : powerlib/Elements/Three-Phase Series RLC Load  Commented=on  LConnTagsString=A|B|C  Configuration=Y (grounded)  NominalVoltage=380  Vabc=[1e3 1e3 1e3]  Vabcp=[1e3 1e3 1e3]  NominalFrequency=50  UnbalancedPower=off  ActivePower=352800  InductivePower=158760  CapacitivePower=0  Pabc=[10e3 9e3 11e3]  QLabc=[100 90 110]  QCabc=[100 90 110]  Pabcp=[10e3 9e3 11e3]  QLabcp=[100 90 110]  QCabcp=[100 90 110]  Measurements=None  LoadType=constant Z
  Three-Phase Series RLC Load1 : powerlib/Elements/Three-Phase Series RLC Load  LConnTagsString=A|B|C  Configuration=Y (grounded)  NominalVoltage=380  Vabc=[1e3 1e3 1e3]  Vabcp=[1e3 1e3 1e3]  NominalFrequency=50  UnbalancedPower=off  ActivePower=0.1*352800  InductivePower=0  CapacitivePower=0  Pabc=[10e3 9e3 11e3]  QLabc=[100 90 110]  QCabc=[100 90 110]  Pabcp=[10e3 9e3 11e3]  QLabcp=[100 90 110]  QCabcp=[100 90 110]  Measurements=None  LoadType=constant Z
  Three-Phase Series RLC Load2 : powerlib/Elements/Three-Phase Series RLC Load  LConnTagsString=A|B|C  Configuration=Y (grounded)  NominalVoltage=380  Vabc=[1e3 1e3 1e3]  Vabcp=[1e3 1e3 1e3]  NominalFrequency=50  UnbalancedPower=off  ActivePower=0.9*352800  InductivePower=158760  CapacitivePower=0  Pabc=[10e3 9e3 11e3]  QLabc=[100 90 110]  QCabc=[100 90 110]  Pabcp=[10e3 9e3 11e3]  QLabcp=[100 90 110]  QCabcp=[100 90 110]  Measurements=None  LoadType=constant Z
  A : PMIOPort  Side=Right
  B : PMIOPort  Port=2  Side=Right
  C : PMIOPort  Port=3  Side=Right
  connections:
  Q/LConn3 -- T/LConn3
  Q/LConn1 -- T/LConn1
  Q/RConn2 -- B/RConn1
  Q/RConn1 -- A/RConn1
  Q/LConn2 -- T/LConn2
  Q/RConn3 -- C/RConn1
  Three-Phase Series RLC Load1/LConn3 -- Three-Phase Series RLC Load2/LConn3 -- Three-Phase Series RLC Load/LConn3 -- Nonlinear Load/LConn3 -- Nonlinear Load 3ph/LConn3 -- T/RConn3 -- Load/LConn3
  Three-Phase Series RLC Load1/LConn2 -- Three-Phase Series RLC Load2/LConn2 -- Three-Phase Series RLC Load/LConn2 -- Nonlinear Load/LConn2 -- Nonlinear Load 3ph/LConn2 -- Load/LConn2 -- T/RConn2
  Three-Phase Series RLC Load2/LConn1 -- Three-Phase Series RLC Load1/LConn1 -- Three-Phase Series RLC Load/LConn1 -- Nonlinear Load/LConn1 -- Nonlinear Load 3ph/LConn1 -- Load/LConn1 -- T/RConn1

== system SPGF_FSK_0000_R2019b/TP43 ==
  Load : powerlib/Elements/Three-Phase Parallel RLC Load  Commented=on  LConnTagsString=A|B|C  Configuration=Y (grounded)  NominalVoltage=380  Vabc=[1e3 1e3 1e3]  Vabcp=[1e3 1e3 1e3]  NominalFrequency=50  UnbalancedPower=off  ActivePower=224000  InductivePower=100800  CapacitivePower=0  Pabc=[10e3 9e3 11e3]  QLabc=[100 90 110]  QCabc=[100 90 110]  Pabcp=[10e3 9e3 11e3]  QLabcp=[100 90 110]  QCabcp=[100 90 110]  Measurements=None  LoadType=constant PQ
  Nonlinear Load : Subsystem  Commented=on
  Nonlinear Load 3ph : Subsystem
  Q : Subsystem
  T : powerlib/Elements/Three-Phase Transformer (Two Windings)  Winding1Connection=Y  Winding2Connection=Yg  CoreType=Three single-phase transformers  SetSaturation=on  Hysteresis=off  DataFile='hysteresis'  SetInitialFlux=off  Measurements=None  UNITS=pu  NominalPower=[400000, 50]  Winding1=[10250, 0.00687500, 0.02250000]  Winding2=[400.00, 0.00687500, 0.02250000]  Rm=444.444  Lm=55.5556  L0=2  Saturation=[0 0;0.01774 0.324129;0.0487637 0.61284;0.0980856 0.825118;0.2 1;0.309543 1.08024;0.652348 1.17344;2.0357 1.26115;6.0215 1.36094;12.4388 1.49469]  InitialFluxes=[-0.920672603859646 0.0224556996452308 0.898216904214336]  BreakLoop=on  DiscreteSolver=Trapezoidal iterative  DataType=off  TransfoNumber=1
  Three-Phase Series RLC Load : powerlib/Elements/Three-Phase Series RLC Load  Commented=on  LConnTagsString=A|B|C  Configuration=Y (grounded)  NominalVoltage=380  Vabc=[1e3 1e3 1e3]  Vabcp=[1e3 1e3 1e3]  NominalFrequency=50  UnbalancedPower=off  ActivePower=224000  InductivePower=100800  CapacitivePower=0  Pabc=[10e3 9e3 11e3]  QLabc=[100 90 110]  QCabc=[100 90 110]  Pabcp=[10e3 9e3 11e3]  QLabcp=[100 90 110]  QCabcp=[100 90 110]  Measurements=None  LoadType=constant Z
  Three-Phase Series RLC Load1 : powerlib/Elements/Three-Phase Series RLC Load  LConnTagsString=A|B|C  Configuration=Y (grounded)  NominalVoltage=380  Vabc=[1e3 1e3 1e3]  Vabcp=[1e3 1e3 1e3]  NominalFrequency=50  UnbalancedPower=off  ActivePower=0.1*224000  InductivePower=0  CapacitivePower=0  Pabc=[10e3 9e3 11e3]  QLabc=[100 90 110]  QCabc=[100 90 110]  Pabcp=[10e3 9e3 11e3]  QLabcp=[100 90 110]  QCabcp=[100 90 110]  Measurements=None  LoadType=constant Z
  Three-Phase Series RLC Load2 : powerlib/Elements/Three-Phase Series RLC Load  LConnTagsString=A|B|C  Configuration=Y (grounded)  NominalVoltage=380  Vabc=[1e3 1e3 1e3]  Vabcp=[1e3 1e3 1e3]  NominalFrequency=50  UnbalancedPower=off  ActivePower=0.9*224000  InductivePower=100800  CapacitivePower=0  Pabc=[10e3 9e3 11e3]  QLabc=[100 90 110]  QCabc=[100 90 110]  Pabcp=[10e3 9e3 11e3]  QLabcp=[100 90 110]  QCabcp=[100 90 110]  Measurements=None  LoadType=constant Z
  A : PMIOPort  Side=Right
  B : PMIOPort  Port=2  Side=Right
  C : PMIOPort  Port=3  Side=Right
  connections:
  Three-Phase Series RLC Load2/LConn1 -- Three-Phase Series RLC Load1/LConn1 -- Three-Phase Series RLC Load/LConn1 -- Nonlinear Load/LConn1 -- Nonlinear Load 3ph/LConn1 -- Load/LConn1 -- T/RConn1
  Three-Phase Series RLC Load2/LConn2 -- Three-Phase Series RLC Load1/LConn2 -- Three-Phase Series RLC Load/LConn2 -- Nonlinear Load/LConn2 -- Nonlinear Load 3ph/LConn2 -- Load/LConn2 -- T/RConn2
  Three-Phase Series RLC Load2/LConn3 -- Three-Phase Series RLC Load1/LConn3 -- Three-Phase Series RLC Load/LConn3 -- Nonlinear Load/LConn3 -- Nonlinear Load 3ph/LConn3 -- T/RConn3 -- Load/LConn3
  Q/RConn3 -- C/RConn1
  Q/LConn2 -- T/LConn2
  Q/RConn1 -- A/RConn1
  Q/RConn2 -- B/RConn1
  Q/LConn1 -- T/LConn1
  Q/LConn3 -- T/LConn3

== system SPGF_FSK_0000_R2019b/TP51 ==
  Load : powerlib/Elements/Three-Phase Parallel RLC Load  Commented=on  LConnTagsString=A|B|C  Configuration=Y (grounded)  NominalVoltage=380  Vabc=[1e3 1e3 1e3]  Vabcp=[1e3 1e3 1e3]  NominalFrequency=50  UnbalancedPower=off  ActivePower=224000  InductivePower=100800  CapacitivePower=0  Pabc=[10e3 9e3 11e3]  QLabc=[100 90 110]  QCabc=[100 90 110]  Pabcp=[10e3 9e3 11e3]  QLabcp=[100 90 110]  QCabcp=[100 90 110]  Measurements=None  LoadType=constant PQ
  Nonlinear Load : Subsystem  Commented=on
  Nonlinear Load 3ph : Subsystem
  Q : Subsystem
  T : powerlib/Elements/Three-Phase Transformer (Two Windings)  Winding1Connection=Y  Winding2Connection=Yg  CoreType=Three single-phase transformers  SetSaturation=on  Hysteresis=off  DataFile='hysteresis'  SetInitialFlux=off  Measurements=None  UNITS=pu  NominalPower=[400000, 50]  Winding1=[10250, 0.00687500, 0.02250000]  Winding2=[400.00, 0.00687500, 0.02250000]  Rm=444.444  Lm=55.5556  L0=2  Saturation=[0 0;0.01774 0.324129;0.0487637 0.61284;0.0980856 0.825118;0.2 1;0.309543 1.08024;0.652348 1.17344;2.0357 1.26115;6.0215 1.36094;12.4388 1.49469]  InitialFluxes=[-0.920724540873851 0.0226319899806901 0.898092550893189]  BreakLoop=on  DiscreteSolver=Trapezoidal iterative  DataType=off  TransfoNumber=1
  Three-Phase Series RLC Load : powerlib/Elements/Three-Phase Series RLC Load  Commented=on  LConnTagsString=A|B|C  Configuration=Y (grounded)  NominalVoltage=380  Vabc=[1e3 1e3 1e3]  Vabcp=[1e3 1e3 1e3]  NominalFrequency=50  UnbalancedPower=off  ActivePower=224000  InductivePower=100800  CapacitivePower=0  Pabc=[10e3 9e3 11e3]  QLabc=[100 90 110]  QCabc=[100 90 110]  Pabcp=[10e3 9e3 11e3]  QLabcp=[100 90 110]  QCabcp=[100 90 110]  Measurements=None  LoadType=constant Z
  Three-Phase Series RLC Load1 : powerlib/Elements/Three-Phase Series RLC Load  LConnTagsString=A|B|C  Configuration=Y (grounded)  NominalVoltage=380  Vabc=[1e3 1e3 1e3]  Vabcp=[1e3 1e3 1e3]  NominalFrequency=50  UnbalancedPower=off  ActivePower=0.1*224000  InductivePower=0  CapacitivePower=0  Pabc=[10e3 9e3 11e3]  QLabc=[100 90 110]  QCabc=[100 90 110]  Pabcp=[10e3 9e3 11e3]  QLabcp=[100 90 110]  QCabcp=[100 90 110]  Measurements=None  LoadType=constant Z
  Three-Phase Series RLC Load2 : powerlib/Elements/Three-Phase Series RLC Load  LConnTagsString=A|B|C  Configuration=Y (grounded)  NominalVoltage=380  Vabc=[1e3 1e3 1e3]  Vabcp=[1e3 1e3 1e3]  NominalFrequency=50  UnbalancedPower=off  ActivePower=0.9*224000  InductivePower=100800  CapacitivePower=0  Pabc=[10e3 9e3 11e3]  QLabc=[100 90 110]  QCabc=[100 90 110]  Pabcp=[10e3 9e3 11e3]  QLabcp=[100 90 110]  QCabcp=[100 90 110]  Measurements=None  LoadType=constant Z
  A : PMIOPort  Side=Right
  B : PMIOPort  Port=2  Side=Right
  C : PMIOPort  Port=3  Side=Right
  connections:
  Three-Phase Series RLC Load2/LConn1 -- Three-Phase Series RLC Load1/LConn1 -- Three-Phase Series RLC Load/LConn1 -- Nonlinear Load/LConn1 -- Nonlinear Load 3ph/LConn1 -- Load/LConn1 -- T/RConn1
  Three-Phase Series RLC Load2/LConn2 -- Three-Phase Series RLC Load1/LConn2 -- Three-Phase Series RLC Load/LConn2 -- Nonlinear Load/LConn2 -- Nonlinear Load 3ph/LConn2 -- Load/LConn2 -- T/RConn2
  Three-Phase Series RLC Load1/LConn3 -- Three-Phase Series RLC Load2/LConn3 -- Three-Phase Series RLC Load/LConn3 -- Nonlinear Load/LConn3 -- Nonlinear Load 3ph/LConn3 -- T/RConn3 -- Load/LConn3
  Q/RConn3 -- C/RConn1
  Q/LConn2 -- T/LConn2
  Q/RConn1 -- A/RConn1
  Q/RConn2 -- B/RConn1
  Q/LConn1 -- T/LConn1
  Q/LConn3 -- T/LConn3

== system SPGF_FSK_0000_R2019b/TP52 ==
  Load : powerlib/Elements/Three-Phase Parallel RLC Load  Commented=on  LConnTagsString=A|B|C  Configuration=Y (grounded)  NominalVoltage=380  Vabc=[1e3 1e3 1e3]  Vabcp=[1e3 1e3 1e3]  NominalFrequency=50  UnbalancedPower=off  ActivePower=560000  InductivePower=252000  CapacitivePower=0  Pabc=[10e3 9e3 11e3]  QLabc=[100 90 110]  QCabc=[100 90 110]  Pabcp=[10e3 9e3 11e3]  QLabcp=[100 90 110]  QCabcp=[100 90 110]  Measurements=None  LoadType=constant PQ
  Nonlinear Load : Subsystem  Commented=on
  Nonlinear Load 3ph : Subsystem
  Q : Subsystem
  T : powerlib/Elements/Three-Phase Transformer (Two Windings)  Winding1Connection=Y  Winding2Connection=Yg  CoreType=Three single-phase transformers  SetSaturation=on  Hysteresis=off  DataFile='hysteresis'  SetInitialFlux=off  Measurements=None  UNITS=pu  NominalPower=[1000000, 50]  Winding1=[10250, 0.00610000, 0.02750000]  Winding2=[400.00, 0.00610000, 0.02750000]  Rm=526.316  Lm=58.8235  L0=2  Saturation=[0 0;0.01774 0.324129;0.0487637 0.61284;0.0980856 0.825118;0.2 1;0.309543 1.08024;0.652348 1.17344;2.0357 1.26115;6.0215 1.36094;12.4388 1.49469]  InitialFluxes=[-0.919410914471537 0.0255116004444432 0.893899314027097]  BreakLoop=on  DiscreteSolver=Trapezoidal iterative  DataType=off  TransfoNumber=1
  Three-Phase Series RLC Load : powerlib/Elements/Three-Phase Series RLC Load  Commented=on  LConnTagsString=A|B|C  Configuration=Y (grounded)  NominalVoltage=380  Vabc=[1e3 1e3 1e3]  Vabcp=[1e3 1e3 1e3]  NominalFrequency=50  UnbalancedPower=off  ActivePower=560000  InductivePower=252000  CapacitivePower=0  Pabc=[10e3 9e3 11e3]  QLabc=[100 90 110]  QCabc=[100 90 110]  Pabcp=[10e3 9e3 11e3]  QLabcp=[100 90 110]  QCabcp=[100 90 110]  Measurements=None  LoadType=constant Z
  Three-Phase Series RLC Load1 : powerlib/Elements/Three-Phase Series RLC Load  LConnTagsString=A|B|C  Configuration=Y (grounded)  NominalVoltage=380  Vabc=[1e3 1e3 1e3]  Vabcp=[1e3 1e3 1e3]  NominalFrequency=50  UnbalancedPower=off  ActivePower=0.1*560000  InductivePower=0  CapacitivePower=0  Pabc=[10e3 9e3 11e3]  QLabc=[100 90 110]  QCabc=[100 90 110]  Pabcp=[10e3 9e3 11e3]  QLabcp=[100 90 110]  QCabcp=[100 90 110]  Measurements=None  LoadType=constant Z
  Three-Phase Series RLC Load2 : powerlib/Elements/Three-Phase Series RLC Load  LConnTagsString=A|B|C  Configuration=Y (grounded)  NominalVoltage=380  Vabc=[1e3 1e3 1e3]  Vabcp=[1e3 1e3 1e3]  NominalFrequency=50  UnbalancedPower=off  ActivePower=0.9*560000  InductivePower=252000  CapacitivePower=0  Pabc=[10e3 9e3 11e3]  QLabc=[100 90 110]  QCabc=[100 90 110]  Pabcp=[10e3 9e3 11e3]  QLabcp=[100 90 110]  QCabcp=[100 90 110]  Measurements=None  LoadType=constant Z
  A : PMIOPort  Side=Right
  B : PMIOPort  Port=2  Side=Right
  C : PMIOPort  Port=3  Side=Right
  connections:
  Q/LConn3 -- T/LConn3
  Q/LConn1 -- T/LConn1
  Q/RConn2 -- B/RConn1
  Q/RConn1 -- A/RConn1
  Q/LConn2 -- T/LConn2
  Q/RConn3 -- C/RConn1
  Three-Phase Series RLC Load1/LConn3 -- Three-Phase Series RLC Load2/LConn3 -- Nonlinear Load/LConn3 -- Nonlinear Load 3ph/LConn3 -- T/RConn3 -- Load/LConn3 -- Three-Phase Series RLC Load/LConn3
  Three-Phase Series RLC Load1/LConn2 -- Three-Phase Series RLC Load2/LConn2 -- Nonlinear Load/LConn2 -- Nonlinear Load 3ph/LConn2 -- Load/LConn2 -- T/RConn2 -- Three-Phase Series RLC Load/LConn2
  Three-Phase Series RLC Load/LConn1 -- Nonlinear Load/LConn1 -- Nonlinear Load 3ph/LConn1 -- T/RConn1 -- Load/LConn1 -- Three-Phase Series RLC Load2/LConn1 -- Three-Phase Series RLC Load1/LConn1

== system SPGF_FSK_0000_R2019b/TP53 ==
  Load : powerlib/Elements/Three-Phase Parallel RLC Load  Commented=on  LConnTagsString=A|B|C  Configuration=Y (grounded)  NominalVoltage=380  Vabc=[1e3 1e3 1e3]  Vabcp=[1e3 1e3 1e3]  NominalFrequency=50  UnbalancedPower=off  ActivePower=224000  InductivePower=100800  CapacitivePower=0  Pabc=[10e3 9e3 11e3]  QLabc=[100 90 110]  QCabc=[100 90 110]  Pabcp=[10e3 9e3 11e3]  QLabcp=[100 90 110]  QCabcp=[100 90 110]  Measurements=None  LoadType=constant PQ
  Nonlinear Load : Subsystem  Commented=on
  Nonlinear Load 3ph : Subsystem
  Q : Subsystem
  T : powerlib/Elements/Three-Phase Transformer (Two Windings)  Winding1Connection=Y  Winding2Connection=Yg  CoreType=Three single-phase transformers  SetSaturation=on  Hysteresis=off  DataFile='hysteresis'  SetInitialFlux=off  Measurements=None  UNITS=pu  NominalPower=[400000, 50]  Winding1=[10250, 0.00687500, 0.02250000]  Winding2=[400.00, 0.00687500, 0.02250000]  Rm=444.444  Lm=55.5556  L0=2  Saturation=[0 0;0.01774 0.324129;0.0487637 0.61284;0.0980856 0.825118;0.2 1;0.309543 1.08024;0.652348 1.17344;2.0357 1.26115;6.0215 1.36094;12.4388 1.49469]  InitialFluxes=[-0.918580759415888 0.0221773071272597 0.896403452288678]  BreakLoop=on  DiscreteSolver=Trapezoidal iterative  DataType=off  TransfoNumber=1
  Three-Phase Series RLC Load : powerlib/Elements/Three-Phase Series RLC Load  Commented=on  LConnTagsString=A|B|C  Configuration=Y (grounded)  NominalVoltage=380  Vabc=[1e3 1e3 1e3]  Vabcp=[1e3 1e3 1e3]  NominalFrequency=50  UnbalancedPower=off  ActivePower=224000  InductivePower=100800  CapacitivePower=0  Pabc=[10e3 9e3 11e3]  QLabc=[100 90 110]  QCabc=[100 90 110]  Pabcp=[10e3 9e3 11e3]  QLabcp=[100 90 110]  QCabcp=[100 90 110]  Measurements=None  LoadType=constant Z
  Three-Phase Series RLC Load1 : powerlib/Elements/Three-Phase Series RLC Load  LConnTagsString=A|B|C  Configuration=Y (grounded)  NominalVoltage=380  Vabc=[1e3 1e3 1e3]  Vabcp=[1e3 1e3 1e3]  NominalFrequency=50  UnbalancedPower=off  ActivePower=0.1*224000  InductivePower=0  CapacitivePower=0  Pabc=[10e3 9e3 11e3]  QLabc=[100 90 110]  QCabc=[100 90 110]  Pabcp=[10e3 9e3 11e3]  QLabcp=[100 90 110]  QCabcp=[100 90 110]  Measurements=None  LoadType=constant Z
  Three-Phase Series RLC Load2 : powerlib/Elements/Three-Phase Series RLC Load  LConnTagsString=A|B|C  Configuration=Y (grounded)  NominalVoltage=380  Vabc=[1e3 1e3 1e3]  Vabcp=[1e3 1e3 1e3]  NominalFrequency=50  UnbalancedPower=off  ActivePower=0.9*224000  InductivePower=100800  CapacitivePower=0  Pabc=[10e3 9e3 11e3]  QLabc=[100 90 110]  QCabc=[100 90 110]  Pabcp=[10e3 9e3 11e3]  QLabcp=[100 90 110]  QCabcp=[100 90 110]  Measurements=None  LoadType=constant Z
  A : PMIOPort  Side=Right
  B : PMIOPort  Port=2  Side=Right
  C : PMIOPort  Port=3  Side=Right
  connections:
  Three-Phase Series RLC Load1/LConn1 -- Three-Phase Series RLC Load2/LConn1 -- Three-Phase Series RLC Load/LConn1 -- Nonlinear Load/LConn1 -- Nonlinear Load 3ph/LConn1 -- T/RConn1 -- Load/LConn1
  Three-Phase Series RLC Load2/LConn2 -- Three-Phase Series RLC Load1/LConn2 -- Three-Phase Series RLC Load/LConn2 -- Nonlinear Load/LConn2 -- Nonlinear Load 3ph/LConn2 -- T/RConn2 -- Load/LConn2
  Three-Phase Series RLC Load2/LConn3 -- Three-Phase Series RLC Load1/LConn3 -- Three-Phase Series RLC Load/LConn3 -- Nonlinear Load/LConn3 -- Nonlinear Load 3ph/LConn3 -- T/RConn3 -- Load/LConn3
  Q/RConn3 -- C/RConn1
  Q/LConn2 -- T/LConn2
  Q/RConn1 -- A/RConn1
  Q/RConn2 -- B/RConn1
  Q/LConn1 -- T/LConn1
  Q/LConn3 -- T/LConn3
